simulink model "test_formation"  (R2025b)
settings: Solver=ode4  StartTime=0.0  StopTime=500  FixedStep=0.01  RelTol=1e-3
libraries: simulink_extras x9
(part 3 of 3)

== matlab function test_formation/Subsystem/Synthesize Commands/Augemented Cucker Smale Model/Alignment ==
  data: agent input; align output
function align = ACS(agent)
%% Params
idx         = 1; % Agent ID
lamda       = 1; % Alignment Strength
beta        = 0.25; % Communication Decay rate
N           = size(agent, 2); % The number of Agents
align       = zeros(3, 1); % Initialize Output
sum_acc     = zeros(3,1);

%% Formation pattern parameters
l = [1/sqrt(2) 1/sqrt(2) 0]';
gamma = 2;


%% Agent_i Information
pos_i       = agent(1:3, idx); % Position
vel_i       = agent(4:6, idx); % Velocity

total_pos = zeros(3,1);
for i = 1:N
    total_pos = total_pos + agent(1:3,i);
end
avg_pos = total_pos/N;
% F = gamma * [ &lt;xi - x_bar, l&gt; * l - (xi - x_bar) ]
relative_pos = pos_i - avg_pos;           % xi - x_bar
projection = dot(relative_pos, l) * l;    % &lt;xi - x_bar, l&gt; * l
F = gamma * (projection - relative_pos);  % 직선 방향으로 끌어당기는 힘


%% Skip calculation if there are fewer than two agents.
if N < 2
    return;
end

%% Algorithm.
for j = 1 : N
    if j ==idx
        continue ;
    end

    % Jth Identification. 
    pos_j   = agent(1:3, j);
    vel_j   = agent(4:6, j);

    r_ij    = norm(pos_i - pos_j);
    psi     = 1 / (1+r_ij^2)^beta;
    vel     = vel_j - vel_i;
    sum_acc = sum_acc + psi*vel;    
end

%% Output (Virtual Control Input)
align       = (lamda/N*sum_acc)+F;

== matlab function test_formation/Subsystem1/Synthesize Commands/Vector Field Guidance/MATLAB Function ==
  data: state input; VFG output; psi_wrapped output; des_psi output; psi_err output
function [VFG,psi_wrapped ,des_psi, psi_err] = fcn(state)
%% 1. State Input (Inertial Frame)
x = state(1);
y = state(2);
z = state(3);
V = state(4);      % Airspeed (or Groundspeed)
gam = state(5);    % Flight path angle
psi = state(6);    % Heading angle
% psi = atan2(sin(psi), cos(psi));
% des_psi = psi;
%% 2. Parameters
xt = 0; yt = 0; zt = -100; % Target Position (NED 기준, -100m는 상공)
Vd = 20;                   % Desired Speed
rd = 500;                  % Desired Orbit Radius

%% 3. Desired Velocity Vector Field (Equation 7)
xr = x - xt;
yr = y - yt;
r = sqrt(xr^2 + yr^2);

% 분모 0 방지 및 수치 안정성 확보
r_safe = max(r, 0.01);

% Matrix A &amp; B formulation (Equation 7)
% 논문의 수식: [xr(r^2-rd^2) + yr(2r rd); yr(r^2-rd^2) - xr(2r rd)]
% A = [ (r_safe^2 - rd^2),   (2 * r_safe * rd); 
%      -(2 * r_safe * rd),   (r_safe^2 - rd^2) ];
% B = [xr; yr];

xy_dot = [ 
    (r_safe^2 - rd^2)*xr + (2*r_safe*rd)*yr ;
    (r_safe^2 - rd^2)*yr - (2*r_safe*rd)*xr
    ];

% xy_dot_des = [dot_x_di; dot_y_di]
xy_dot_des = -(Vd / (r_safe * (r_safe^2 + rd^2))) .* xy_dot;

%% 4. Desired Heading Angle (Equation 8)
des_psi = atan2(xy_dot_des(2), xy_dot_des(1));
psi_wrapped = atan2(sin(psi), cos(psi));
%% 5. Control Commands in Horizontally Body-fixed Frame (Equation 5)


% U2: Heading tracking (Lateral) - Angle Wrap-around 처리 필수
% psi_err = des_psi - psi;
% psi_err = atan2(sin(des_psi - psi), cos(des_psi - psi));

% 목표와 현재 각도의 차이 구하기
psi_err = des_psi - psi_wrapped;
% [중요] Reddit 로직: 180도(pi)를 넘어가면 반대 방향 최단거리로 보정
if psi_err > pi
    psi_err = psi_err - 2*pi;
elseif psi_err < -pi
    psi_err = psi_err + 2*pi;
end


U1 = Vd - V * cos(gam); % U1: Speed tracking (Longitudinal)
U2 = V * 1.0*psi_err;
U3 = zt - z; % U3: Altitude tracking (Vertical)
U = [U1; U2; U3];

%% 6. Transform to Inertial Frame (Equation 6)
% R_psi rotation matrix
tran = [
    cos(psi) -sin(psi) 0;
    sin(psi)  cos(psi) 0;
    0         0        1
    ];


% 가속도(또는 속도 변화율) 명령 생성
VFG = tran * U;

== matlab function test_formation/Subsystem/Synthesize Commands/Potential Field/Potential Field ==
  data: agents input; u_pf output
function u_pf = PF(agents)

    %% params
    idx = 1;
    N = size(agents,2);
    alp = 5*sqrt(2); % Potential Strength
    % Bell Function Constant (a, b, c)
    a   = 75; 
    b   = 4;
    c   = 0;
    sum = zeros(3,1);

    % Agent Information
    pos_i = agents(1:3,idx);

    for j = 1: N
        if idx==j 
            continue; 
        end
        pos_j = agents(1:3, j);
        pos_ij = pos_i - pos_j;
        norm_ij = norm(pos_ij);

        val = (norm_ij - c)/a;
        denominator = 1 + (abs(val))^(2*b);
        if norm_ij > 0.001
            sum = sum + (alp/denominator)*(pos_ij/norm_ij);
        end
    end
    u_pf = sum;
end

== matlab function test_formation/Subsystem/Synthesize Commands/Augemented Cucker Smale Model/Repulsion ==
  data: agent input; rep output
function rep = BondingForce2(agent)
    idx     = 1;
    N       = size(agent, 2);
    R       = 75;
    K2      = 0.5; % Bonding gain 2
    pos_i   = agent(1:3, idx);
    acc     = zeros(3,1);
    
    for j = 1:N
        if j == idx, continue; end

        pos_j   = agent(1:3, j);
        r_ij    = norm(pos_i - pos_j);

        if r_ij < 1e-3, r_ij = 1e-3; end
        
        % 2R(150m) 간격을 유지하도록 미는 힘/당기는 힘 계산
        acc     = acc + (K2 / (2 * r_ij)) * (r_ij - 2*R) * (pos_j - pos_i);
    end
    rep         = acc;
end

== matlab function test_formation/Subsystem1/Synthesize Commands/Augemented Cucker Smale Model/Alignment ==
  data: agent input; align output
function align = ACS(agent)
%% Params
idx         = 2; % Agent ID
lamda       = 1; % Alignment Strength
beta        = 0.25; % Communication Decay rate
N           = size(agent, 2); % The number of Agents
align       = zeros(3, 1); % Initialize Output
sum_acc     = zeros(3, 1);

%% Formation pattern parameters
l = [1/sqrt(2) 1/sqrt(2) 0]';
gamma = 2;


%% Agent_i Information
pos_i       = agent(1:3, idx); % Position
vel_i       = agent(4:6, idx); % Velocity

total_pos = zeros(3, 1);
for i = 1:N
    total_pos = total_pos + agent(1:3,i);
end
avg_pos = total_pos/N;
% F = gamma * [ &lt;xi - x_bar, l&gt; * l - (xi - x_bar) ]
relative_pos = pos_i - avg_pos;           % xi - x_bar
projection = dot(relative_pos, l) * l;    % &lt;xi - x_bar, l&gt; * l
F = gamma * (projection - relative_pos);  % 직선 방향으로 끌어당기는 힘


%% Skip calculation if there are fewer than two agents.
if N < 2
    return;
end

%% Algorithm.
for j = 1 : N
    if j ==idx
        continue ;
    end

    % Jth Identification. 
    pos_j   = agent(1:3, j);
    vel_j   = agent(4:6, j);

    r_ij    = norm(pos_i - pos_j);
    psi     = 1 / (1+r_ij^2)^beta;
    vel     = vel_j - vel_i;
    sum_acc = sum_acc + psi*vel;    
end

%% Output (Virtual Control Input)
align       = (lamda/N*sum_acc)+F;




% function align = ACS(agent)
% %% Params
% idx         = 2; % Agent ID
% N           = size(agent, 2); % The number of Agents
% lamda       = 1; % Alignment Strength
% beta        = 0.25; % Communication Decay rate
% align       = zeros(3, 1); % Initialize Output
% sum_acc     = zeros(3,1);
% 
% %% Agent_i Information
% pos_i       = agent(1:3, idx); % Position
% vel_i       = agent(4:6, idx); % Velocity
% 
% %% Skip calculation if there are fewer than two agents.
% if N < 2
%     return;
% end
% 
% %% Algorithm.
% for j = 1 : N
%     if j ==idx
%         continue ;
%     end
% 
%     % Jth Identification. 
%     pos_j   = agent(1:3, j);
%     vel_j   = agent(4:6, j);
% 
%     r_ij    = norm(pos_i - pos_j);
%     psi     = 1 / (1+r_ij^2)^beta;
%     vel     = vel_j - vel_i;
%     sum_acc = sum_acc + psi*vel;    
% end
% 
% %% Output (Virtual Control Input)
% align = lamda/N*sum_acc;
%
